simulink model "arm_test"  (R2023a)
settings: Solver=VariableStepAuto  StartTime=0.0  StopTime=0.5  RelTol=1e-3
settings Model: Creator=LJL  LastModifiedBy=LJL

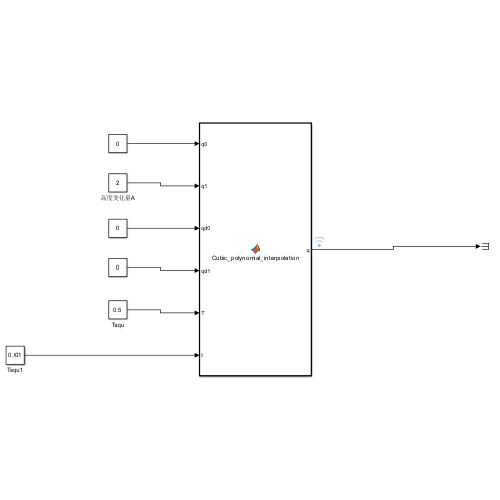
[thumbnail: Simulink's stored preview of the top-level diagram]
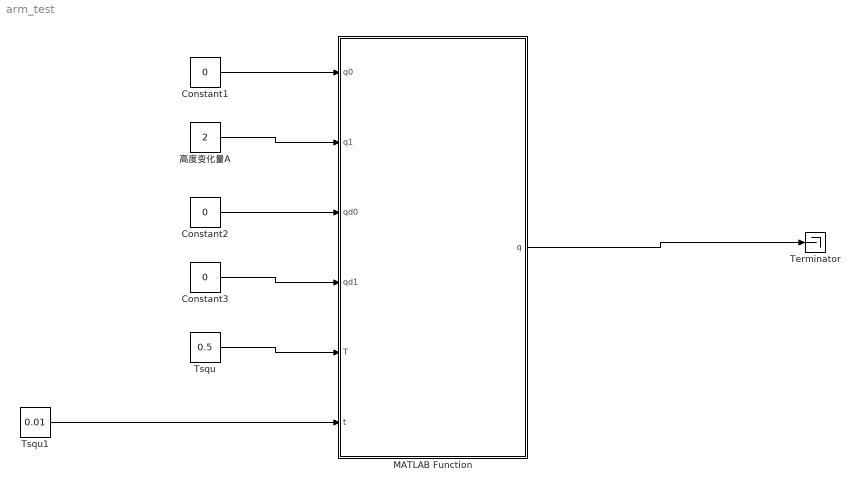
== system arm_test ==
  Constant1 : Constant  Value=0
  Constant2 : Constant  Value=0
  Constant3 : Constant  Value=0
  MATLAB Function : MATLAB Function  TreatAsAtomicUnit=on
  Terminator : Terminator
  Tsqu : Constant  Value=0.5
  Tsqu1 : Constant  Value=0.01
  高度变化量A : Constant  Value=2
  wires:
  Constant3/1 -> MATLAB Function/4(qd1)
  高度变化量A/1 -> MATLAB Function/2(q1)
  Constant1/1 -> MATLAB Function/1(q0)
  Constant2/1 -> MATLAB Function/3(qd0)
  MATLAB Function/1(q) -> Terminator/1
  Tsqu/1 -> MATLAB Function/5(T)
  Tsqu1/1 -> MATLAB Function/6(t)

== matlab function arm_test/MATLAB Function ==
  data: q0 input; q output; q1 input; qd0 input; qd1 input; T input; t input
function q  = Cubic_polynomial_interpolation(q0, q1, qd0, qd1, T, t)
    % 给定初末位置、速度、总时间，返回三次插值后，在时间t（0<t<T）的位置、速度、加速度，t也可以是时间序列
    A = [  0  ,  0 , 0, 1;
         T^3  , T^2, T, 1;
         0    ,  0 , 1, 0;
         3*T^2, 2*T, 1, 0];
    
    B = [q0; q1; qd0; qd1];
    
    % 求解系数矩阵
    p = A \ B;

    % 计算位置、速度、加速度
    q = p(1, :)' * t.^3 + p(2, :)' * t.^2 + p(3, :)' * t + p(4, :)';
    qd = 3 * p(1, :)' * t.^2 + 2 * p(2, :)' * t + p(3, :)';
    qdd = 6 * p(1, :)' * t + 2 * p(2, :)';

end
